simulink model "spectral_averaging"  (R2024a)
settings: Solver=VariableStepAuto  StartTime=0.0  StopTime=2*Nfft/Fs*(Navg-1)  RelTol=1e-3
PreLoadFcn:
  | Navg = 100;
  | Nfft = 1000;
  | Fs = 1e6;
InitFcn:
  | Navg = 100;
  | Nfft = 1000;
  | Fs = 1e6;
StopFcn:
  | post_process_logged_spectrum
undefined symbols (not defined in the file or in its folder): dfilt, dspblkspectrumestimator
libraries: dspsrcs4 x2, dspobslib x1
settings Model: Creator=kschutz  LastModifiedBy=kschutz

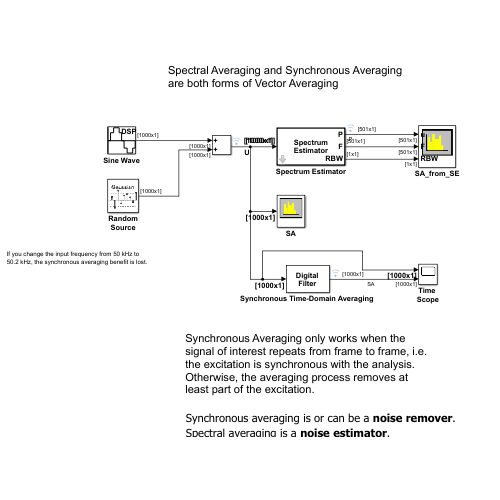
[thumbnail: Simulink's stored preview of the top-level diagram]
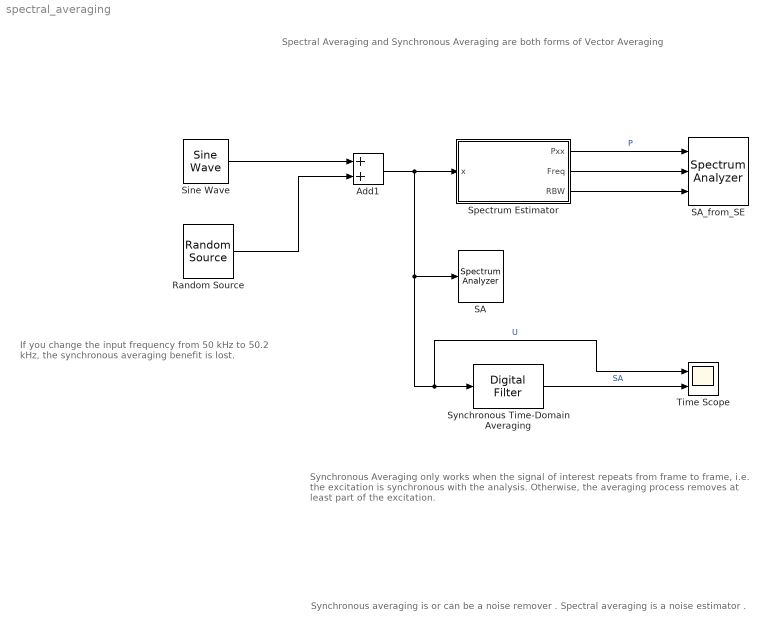
== system spectral_averaging ==
  note: If you change the input frequency from 50 kHz to
      | 50.2 kHz, the synchronous averaging benefit is lost.
  note: Synchronous averaging is or can be a noise remover .
      | Spectral averaging is a noise estimator .
  note: Synchronous Averaging only works when the signal of interest repeats from frame to frame, i.e. the excitation is synchronous with the analysis.
      | Otherwise, the averaging process removes at least part of the excitation.
  note: Spectral Averaging and Synchronous Averaging are both forms of Vector Averaging
  Add1 : Sum
  Random Source : dspsrcs4/Random Source  SrcType=Gaussian  MinVal=0  MaxVal=1  MeanVal=0  VarVal=1  RepMode=Specify seed  rawSeed=123  IsInherit=off  SampTime=1/Fs  SampFrame=Nfft  OutComplex=Real  DataType=double  SimulateUsing=Interpreted execution
  SA : SpectrumAnalyzer  WindowPosition=[26.000000,51.000000,989.000000,526.000000,]  Visible=on  ScopeFrameLocation=window  Method=Welch  SampleRate=100000000  PlotAsTwoSidedSpectrum=off  AxesScaling=Manual  FrequencyResolutionMethod=Window length  WindowLength=1000  FFTLengthSource=Property  FFTLength=1000  Span=50000000  CenterFrequency=25000000  StartFrequency=0  StopFrequency=50000000  Window=Rectangular  VBWSource=Property  VBW=1  SpectrumUnits=dBW  YLimits=[-35.31827535249315,1.256633097506851]  SelectedToolstripTab=spectrumAnalyzerToolstrip.estimationTab  AllowFFTLengthLessThanSamplesPerUpdate=on
  SA_from_SE : SpectrumAnalyzer  NumInputPorts=3  WindowPosition=[466.000000,282.000000,988.000000,516.000000,]  Visible=on  ScopeFrameLocation=window  InputDomain=Frequency  PlotAsTwoSidedSpectrum=off  RBWSource=Input port  Span=10024875.621890547  StartFrequency=-5012437.810945273  StopFrequency=5012437.810945273  InputUnits=dBW  FrequencyVectorSource=Input port  SpectrumUnits=Auto  YLimits=[-34.67607203,0.54062467]  SelectedToolstripTab=spectrumAnalyzerToolstrip.spectrumTab
  Sine Wave : dspsrcs4/Sine Wave  Amplitude=1  Frequency=50e3  Phase=0  SampleMode=Discrete  OutComplex=Real  CompMethod=Trigonometric fcn  TableSize=Speed  SampleTime=1/Fs  SamplesPerFrame=Nfft  ResetState=Restart at time zero  OutputFrames=off  dataType=double  wordLen=16  udDataType=sfix(16)  fracBitsMode=Best precision  numFracBits=15  OutDataTypeStr=double  LastOutDataTypeStr=double
  Spectrum Estimator : Subsystem  InitFcn=dspblkspectrumestimator(gcb,'setup')  TreatAsAtomicUnit=on  mask(Spectrum Estimator){Method=Welch, NumTapsPerBand=12, SpectrumType=Power, FrequencyResolutionMethod=Window length, FilterBankResolutionMethod=Auto, RBW=5, WindowMode=Same as input frame length, WindowLength=1024, FrequencyBandsSource=Same as input frame size, FrequencyBands=1024, FFTLengthSource=Property, FFTLength=Nfft, InheritSampleRate=on, SampleRate=44100, Window=Rectangular, SidelobeAttenuation=60, AveragingMethod=Running, SpectralAverages=Navg, ForgettingFactorPort=off, ForgettingFactor=0.9, Overlap=0, ReferenceLoad=1, FrequencyRange=One-sided, PowerUnits=dBW, SimulateUsing=Code generation, OutputMaxHoldSpectrum=off, OutputMinHoldSpectrum=off, OutputFrequencyVector=on, OutputRBW=on}
      mask prompts: Method "dsp:SpectrumEstimation_BlockDialog:Method_MP"; NumTapsPerBand "dsp:SpectrumEstimation_BlockDialog:NumTaps_MP"; SpectrumType "dsp:SpectrumEstimation_BlockDialog:SpectrumType_MP"; FrequencyResolutionMethod "dsp:SpectrumEstimation_BlockDialog:FrequencyResolutionMethod_MP"; FilterBankResolutionMethod "dsp:SpectrumEstimation_BlockDialog:FrequencyResolutionMethod_MP"; RBW "dsp:SpectrumEstimation_BlockDialog:RBW_MP"; WindowMode "dsp:SpectrumEstimation_BlockDialog:WindowMode_MP"; WindowLength "dsp:SpectrumEstimation_BlockDialog:WindowLength_MP"; FrequencyBandsSource "dsp:SpectrumEstimation_BlockDialog:FrequencyBandsSource_MP"; FrequencyBands "dsp:SpectrumEstimation_BlockDialog:FrequencyBands_MP"; FFTLengthSource "dsp:SpectrumEstimation_BlockDialog:FFTLengthSource_MP"; FFTLength "dsp:SpectrumEstimation_BlockDialog:FFTLength_MP"; InheritSampleRate "dsp:SpectrumEstimation_BlockDialog:InheritSampleRate_MP"; SampleRate "dsp:SpectrumEstimation_BlockDialog:SampleRate_MP"; Window "dsp:SpectrumEstimation_BlockDialog:Window_MP"; SidelobeAttenuation "dsp:SpectrumEstimation_BlockDialog:SidelobeAttenuation_MP"; AveragingMethod "dsp:SpectrumEstimation_BlockDialog:AveragingMethod_MP"; SpectralAverages "dsp:SpectrumEstimation_BlockDialog:SpectralAverages_MP"; ForgettingFactorPort "dsp:system:SpectrumEstimatorBase:ForgettingFactorPort_MP"; ForgettingFactor "dsp:system:SpectrumEstimatorBase:ForgettingFactor_MP"; Overlap "dsp:SpectrumEstimation_BlockDialog:Overlap_MP"; ReferenceLoad "dsp:SpectrumEstimation_BlockDialog:ReferenceLoad_MP"; FrequencyRange "dsp:SpectrumEstimation_BlockDialog:FrequencyRange_MP"; PowerUnits "dsp:SpectrumEstimation_BlockDialog:PowerUnits_MP"; SimulateUsing "dsp:SpectrumEstimation_BlockDialog:SimulateUsing_MP"; OutputMaxHoldSpectrum "dsp:system:SpectrumEstimatorBase:OutputMaxHoldSpectrum_MP"; OutputMinHoldSpectrum "dsp:system:SpectrumEstimatorBase:OutputMinHoldSpectrum_MP"; OutputFrequencyVector "dsp:system:SpectrumEstimatorBase:OutputFrequencyVector_MP"; OutputRBW "dsp:system:SpectrumEstimatorBase:OutputRBW_MP"
      mask help: dsp:SpectrumEstimation_BlockDialog:SpectrumEstimator_MaskDesc
      mask init:
      | dspblkspectrumestimator(gcb,'init')
      settings: LibrarySourceBlock=dspspect3/Spectrum Estimator
      mask Help: eval('blocksethelp');
      mask TypeOptions Method: dsp:SpectrumEstimation_BlockDialog:MethodEnum_Welch | dsp:SpectrumEstimation_BlockDialog:MethodEnum_FilterBank
      mask Callback Method: dspblkspectrumestimator(gcb,'dynamic')
      mask TypeOptions SpectrumType: dsp:SpectrumEstimation_BlockDialog:SpectrumTypeEnum_Power | dsp:SpectrumEstimation_BlockDialog:SpectrumTypeEnum_PowerDensity
      mask TypeOptions FrequencyResolutionMethod: dsp:SpectrumEstimation_BlockDialog:Auto | dsp:SpectrumEstimation_BlockDialog:FrequencyResolutionMethodEnum_RBW | dsp:SpectrumEstimation_BlockDialog:FrequencyResolutionMethodEnum_WindowLength
      mask Callback FrequencyResolutionMethod: dspblkspectrumestimator(gcb,'dynamic')
      mask TypeOptions FilterBankResolutionMethod: dsp:SpectrumEstimation_BlockDialog:Auto | dsp:SpectrumEstimation_BlockDialog:FrequencyResolutionMethodEnum_RBW | dsp:SpectrumEstimation_BlockDialog:FrequencyResolutionMethodEnum_NumBands
      mask Callback FilterBankResolutionMethod: dspblkspectrumestimator(gcb,'dynamic')
      mask TypeOptions WindowMode: dsp:SpectrumEstimation_BlockDialog:WindowLengthSourceEnum_SameAsInput | dsp:SpectrumEstimation_BlockDialog:WindowLengthSourceEnum_Dialog
      mask Callback WindowMode: dspblkspectrumestimator(gcb,'dynamic')
      mask TypeOptions FrequencyBandsSource: dsp:SpectrumEstimation_BlockDialog:SameAsInput | dsp:SpectrumEstimation_BlockDialog:Specify
      mask Callback FrequencyBandsSource: dspblkspectrumestimator(gcb,'dynamic')
      mask Callback FrequencyBands: dspblkspectrumestimator(gcb,'dynamic')
      mask TypeOptions FFTLengthSource: dsp:SpectrumEstimation_BlockDialog:Auto | dsp:SpectrumEstimation_BlockDialog:Property
      mask Callback FFTLengthSource: dspblkspectrumestimator(gcb,'dynamic')
      mask Callback InheritSampleRate: dspblkspectrumestimator(gcb,'dynamic')
      mask TypeOptions Window: dsp:SpectrumEstimation_BlockDialog:WindowEnum_Chebyshev | dsp:SpectrumEstimation_BlockDialog:WindowEnum_FlatTop | dsp:SpectrumEstimation_BlockDialog:WindowEnum_Hamming | dsp:SpectrumEstimation_BlockDialog:WindowEnum_Hann | dsp:SpectrumEstimation_BlockDialog:WindowEnum_Kaiser | dsp:SpectrumEstimation_BlockDialog:WindowEnum_Rectangular
      mask Callback Window: dspblkspectrumestimator(gcb,'dynamic')
      mask TypeOptions AveragingMethod: dsp:SpectrumEstimation_BlockDialog:AveragingMethodEnum_Running | dsp:SpectrumEstimation_BlockDialog:AveragingMethodEnum_Exponential
      mask Callback AveragingMethod: dspblkspectrumestimator(gcb,'dynamic')
      mask TypeOptions ForgettingFactorPort: Spectrum Estimator/ForgettingFactorPort
      mask TypeOptions ForgettingFactor: Spectrum Estimator/ForgettingFactor
      mask TypeOptions FrequencyRange: dsp:SpectrumEstimation_BlockDialog:FrequencyRangeEnum_OneSided | dsp:SpectrumEstimation_BlockDialog:FrequencyRangeEnum_TwoSided | dsp:SpectrumEstimation_BlockDialog:FrequencyRangeEnum_Centered
      mask TypeOptions PowerUnits: dsp:SpectrumEstimation_BlockDialog:PowerUnitsEnum_Watts | dsp:SpectrumEstimation_BlockDialog:PowerUnitsEnum_dBm | dsp:SpectrumEstimation_BlockDialog:PowerUnitsEnum_dBW
      mask TypeOptions SimulateUsing: dsp:SpectrumEstimation_BlockDialog:SimulateUsingEnum_CG | dsp:SpectrumEstimation_BlockDialog:SimulateUsingEnum_Interpreted
      mask TypeOptions OutputMaxHoldSpectrum: Spectrum Estimator/OutputMaxHoldSpectrum
      mask TypeOptions OutputMinHoldSpectrum: Spectrum Estimator/OutputMinHoldSpectrum
      mask TypeOptions OutputFrequencyVector: Spectrum Estimator/OutputFrequencyVector
      mask TypeOptions OutputRBW: Spectrum Estimator/OutputRBW
      mask DialogControl MainTab Prompt: dspshared:FixptDialog:main
      mask DialogControl Method Prompt: Method:
      mask DialogControl NumTapsPerBand Prompt: Number of taps per band:
      mask DialogControl SpectrumType Prompt: Spectrum type:
      mask DialogControl FrequencyResolutionMethod Prompt: Frequency resolution method:
      mask DialogControl FilterBankResolutionMethod Prompt: Frequency resolution method:
      mask DialogControl RBW Prompt: RBW (Hz):
      mask DialogControl WindowMode Prompt: Window length source:
      mask DialogControl WindowLength Prompt: Window length:
      mask DialogControl FrequencyBandsSource Prompt: Number of bands source:
      mask DialogControl FrequencyBands Prompt: Number of bands:
      mask DialogControl FFTLengthSource Prompt: FFT length source:
      mask DialogControl FFTLength Prompt: FFT length:
      mask DialogControl InheritSampleRate Prompt: Inherit sample rate from input
      mask DialogControl SampleRate Prompt: Sample rate (Hz):
      mask DialogControl Window Prompt: Window function:
      mask DialogControl SidelobeAttenuation Prompt: Sidelobe attenuation of window (dB):
      mask DialogControl AveragingMethod Prompt: Averaging method:
      mask DialogControl SpectralAverages Prompt: Number of spectral averages:
      mask DialogControl ForgettingFactorPort Prompt: Specify forgetting factor from input port
      mask DialogControl ForgettingFactor Prompt: Forgetting factor:
      mask DialogControl AdvancedTab Prompt: dsp:SpectrumEstimation_BlockDialog:Advanced
      mask DialogControl Overlap Prompt: Window overlap (%):
      mask DialogControl ReferenceLoad Prompt: Reference load (ohms):
      mask DialogControl FrequencyRange Prompt: Frequency range:
      mask DialogControl PowerUnits Prompt: Power units:
      mask DialogControl OutputMaxHoldSpectrum Prompt: Output max-hold spectrum
      mask DialogControl OutputMinHoldSpectrum Prompt: Output min-hold spectrum
      mask DialogControl OutputFrequencyVector Prompt: Output frequency vector
      mask DialogControl OutputRBW Prompt: Output effective RBW
      mask DialogControl SimulateUsing Prompt: Simulate using
      mask Display:
      | fprintf(getString(message('dsp:system:SpectrumEstimatorBase:SpectrumEstimatorIcon')))
      | blk = gcbh;
      | 
      | % Input port names
      | if get_param(blk,'ForgettingFactorPort')=="on"
      |     port_label('input', 1, 'x');
      |     port_label('input', 2, 'lambda');
      | end
      | 
      | % Output port names
      | showName = false;
      | maxHoldPort = 2;
      | 
      | if get_param(blk,'OutputMaxHoldSpectrum')=="on"
      |     port_label('output', maxHoldPort, 'P_max')
      |     minHoldPort = maxHoldPort + 1;
      |     showName = true;
      | else
      |     minHoldPort = maxHoldPort;
      | end
      | 
      | if get_param(blk,'OutputMinHoldSpectrum')=="on"
      |     port_label('output', minHoldPort, 'P_min')
      |     freqPort = minHoldPort + 1;
      |     showName = true;
      | else
      |     freqPort = minHoldPort;
      | end
      | 
      | if get_param(blk,'OutputFrequencyVector')=="on"
      |     port_label('output', freqPort, 'F')
      |     rbwPort = freqPort + 1;
      |     showName = true;
      | else
      |     rbwPort = freqPort;
      | end
      | 
      | if get_param(blk,'OutputRBW')=="on"
      |     port_label('output', rbwPort, 'RBW')
      |     showName = true;
      | end
      | 
      | if showName
      |    port_label('output', 1, 'P')
      | end
  "Synchronous Time-Domain Averaging " : dspobslib/Digital Filter  TypePopup=IIR (poles & zeros)  IIRFiltStruct=Direct form II transposed  AllPoleFiltStruct=Direct form  FIRFiltStruct=Direct form  CoeffSource=Specify via dialog  NumCoeffs=1/Navg  DenCoeffs=[1 1/Navg-1]  BiQuadCoeffs=[1 0.3 0.4 1 0.1 0.2]  LatticeCoeffs=[0.2 0.4]  denIgnore=on  FiltPerSampPopup=One filter per frame  IC=eps  ICnum=0  ICden=0  roundingMode=Floor  overflowMode=off  ScaleValues=1  scaleValueFracLength=14  stageInFracLength=15  stageOutFracLength=15  FilterSource=Specify via dialog  dfiltObjectName=dfilt.dffir([1 2 1])
  Time Scope : Scope  NumInputPorts=2
  wires:
  Add1/1 -> Time Scope/1, "Synchronous Time-Domain Averaging "/1, SA/1, Spectrum Estimator/1(x)  "U"
  Sine Wave/1 -> Add1/1
  Random Source/1 -> Add1/2
  Spectrum Estimator/2(Freq) -> SA_from_SE/2
  Spectrum Estimator/3(RBW) -> SA_from_SE/3
  "Synchronous Time-Domain Averaging "/1 -> Time Scope/2  "SA"
  Spectrum Estimator/1(Pxx) -> SA_from_SE/1  "P"

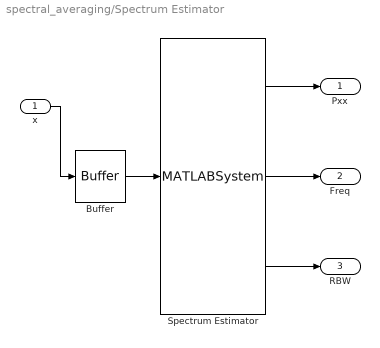
== system spectral_averaging/Spectrum Estimator ==
  x : Inport
  Buffer : Buffer  OutputFrames=off  InheritSize=on  OverlapPercent=Overlap
  Spectrum Estimator : MATLABSystem  System=dsp.simulink.SpectrumEstimator  Method=Welch  NumTapsPerBand=NumTapsPerBand  AveragingMethod=Running  SpectralAverages=100  ForgettingFactorPort=off  ForgettingFactor=ForgettingFactor  FFTLengthSource=Property  FFTLength=1000  AdjustFFTLength=off  Window=Rectangular  SidelobeAttenuation=60  FrequencyRange=onesided  SpectrumType=Power  PowerUnits=dBW  ReferenceLoad=ReferenceLoad  OutputMaxHoldSpectrum=off  OutputMinHoldSpectrum=off  OutputFrequencyVector=on  OutputRBW=on  InheritSampleRate=on  SampleRate=44100  SimulateUsing=Code generation
      mask Type: dsp.simulink.SpectrumEstimator
      mask Display:
      | disp(['Spectrum' char(10) 'Estimator']);
      | port_label('output',1,'P');
      | port_label('output',2,'F');
      | port_label('output',3,'RBW');
  Pxx : Outport  VectorParamsAs1DForOutWhenUnconnected=off
  Freq : Outport  Port=2
  RBW : Outport  Port=3
  wires:
  Spectrum Estimator/1 -> Pxx/1
  x/1 -> Buffer/1
  Buffer/1 -> Spectrum Estimator/1
  Spectrum Estimator/2 -> Freq/1
  Spectrum Estimator/3 -> RBW/1
